simulink model "Voltage_Source_Inverter_fed_Asynchronous_Motor_Drive"  (R2020b)
settings: Solver=VariableStepAuto  StartTime=0.0  StopTime=10  RelTol=1e-3
libraries: powerlib x12, powerlib_meascontrol x1
settings Model: Creator=adima  LastModifiedBy=adima

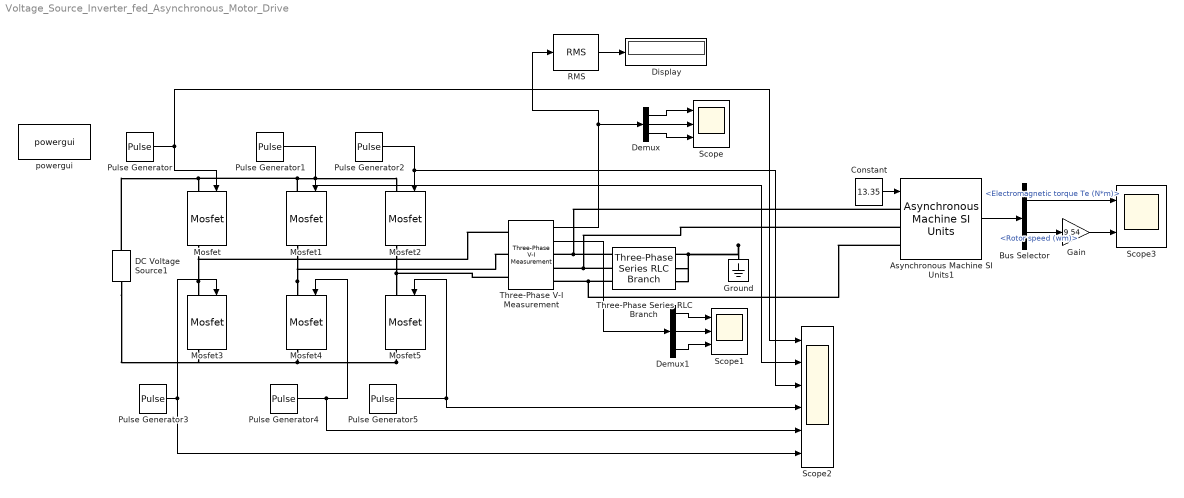
== system Voltage_Source_Inverter_fed_Asynchronous_Motor_Drive ==
  Asynchronous Machine SI Units1 : powerlib/Machines/Asynchronous Machine SI Units  RotorType=Squirrel-cage  PresetModel="15:  5.4 HP (4KW)   400 V  50Hz 1430 RPM"  MechanicalLoad=Torque Tm  ShowDetailedParameters=on  ReferenceFrame=Rotor  Units=SI  MeasurementBus=off  NominalParameters=[4000 400 50]  Stator=[1.405 0.005839]  Rotor=[1.395 0.005839]  Cage1=[0.4155 0.002066]  Cage2=[0.4168 0.0003495]  Lm=0.1722  Mechanical=[0.0131 0.002985 2]  PolePairs=2  InitialConditions=[0 0 0 0 0 0 0 0]  SimulateSaturation=off  Saturation=[14.03593122, 27.81365428, 53.79336849, 72.68890987, 97.98006896, 148.6815601, 215.7428561, 302.9841135, 428.7778367 ; 230, 322, 414, 460, 506, 552, 598, 644, 690]  LoadFlowParameters=1492000  TsPowergui=0  TsBlock=-1  IterativeModel=Trapezoidal non iterative  IterativeDiscreteModel=Trapezoidal non iterative  Pmec=1.492e+006
  Bus Selector : BusSelector  OutputSignals=Mechanical.Electromagnetic torque Te (N*m),Mechanical.Rotor speed (wm)
  Constant : Constant  Value=13.35
  DC Voltage Source1 : powerlib/Electrical Sources/DC Voltage Source  Amplitude=300  Measurements=None
  Demux : Demux  Outputs=3
  Demux1 : Demux  Outputs=3
  Display : Display
  Gain : Gain  Gain=9.54
  Ground : powerlib/Elements/Ground  LConnTagsString=a
  Mosfet{,1..5} (6 alike) : powerlib/Power Electronics/Mosfet  Ron=0.1  Lon=0  Rd=0.01  Vfd=0  IC=0  Rs=1e5  Cs=inf  Measurements=on
  Pulse Generator : DiscretePulseGenerator  PulseType=Time based  Period=1/50  PulseWidth=50
  Pulse Generator1 : DiscretePulseGenerator  PulseType=Time based  Period=1/50  PulseWidth=50  PhaseDelay=120*((20e-3)/360)
  Pulse Generator2 : DiscretePulseGenerator  PulseType=Time based  Period=1/50  PulseWidth=50  PhaseDelay=240*((20e-3)/360)
  Pulse Generator3 : DiscretePulseGenerator  PulseType=Time based  Period=1/50  PulseWidth=50  PhaseDelay=180*((20e-3)/360)
  Pulse Generator4 : DiscretePulseGenerator  PulseType=Time based  Period=1/50  PulseWidth=50  PhaseDelay=300*((20e-3)/360)
  Pulse Generator5 : DiscretePulseGenerator  PulseType=Time based  Period=1/50  PulseWidth=50  PhaseDelay=60*((20e-3)/360)
  RMS : powerlib_meascontrol/Measurements/RMS  TrueRMS=on  Freq=60  RMSInit=120  Ts=0
  Scope : Scope  NumInputPorts=3
  Scope1 : Scope  NumInputPorts=3
  Scope2 : Scope  NumInputPorts=6
  Scope3 : Scope  NumInputPorts=2
  Three-Phase Series RLC Branch : powerlib/Elements/Three-Phase Series RLC Branch  LConnTagsString=A|B|C  RConnTagsString=A|B|C  BranchType=R  Resistance=10  Inductance=1e-3  Capacitance=1e-6  Measurements=None
  Three-Phase V-I Measurement : powerlib/Measurements/Three-Phase V-I Measurement  VoltageMeasurement=phase-to-ground  SetLabelV=off  LabelV=Vabc  Vpu=off  VpuLL=off  CurrentMeasurement=yes  SetLabelI=off  LabelI=Iabc  Ipu=off  Pbase=100e6  Vbase=500e3  OutputType=Complex  PhasorSimulation=off  PSBequivalent=0
  powergui : powerlib/powergui  Priority=1  SimulationMode=Discrete  SampleTime=5e-6  frequency=60  Iterations=50  frequencyindice=0  Pbase=100e6  ErrMax=1e-4  UnitsV=kV  UnitsW=MW  buscounter=0  FunctionMessages=off  echomessages=off  EnableUseOfTLC=off  CurrentSourceSwitches=off  DisableSnubberDevices=off  DisableRonSwitches=off  DisableVfSwitches=off  DisplayEquations=off  AutomaticDiscreteSolvers=off  SolverType=Tustin/Backward Euler (TBE)  Interpol=off  ExternalGateDelay=off  methode=off  Ts=100  x0status=blocks  SPID=on  SwTol=0  HookPort=off  NonlinearTolerance=1e-4  nMaxIteration=100  ContinueOnMaxIteration=off  RestoreLinks=warning  ResistiveCurrentMeasurement=off  Frange=[0:2:500]  Ylog=off  Xlog=on  ShowGrid=off  save=off  variable=ZData  structure=0  ZoomFFT=off  StartTime=0.0  cycles=1  DisplayStyle=1  fundamental=60  FreqAxis=off  MaxFrequency=1000  frequencyindicesteady=1  RmsSteady=1  display=off
  wires:
  Demux1/1 -> Scope1/1
  RMS/1 -> Display/1
  Three-Phase V-I Measurement/2 -> Demux1/1
  Demux/2 -> Scope/2
  Pulse Generator1/1 -> Mosfet1/1, Scope2/2
  Pulse Generator/1 -> Mosfet/1, Scope2/1
  Pulse Generator2/1 -> Scope2/3, Mosfet2/1
  Pulse Generator4/1 -> Scope2/5, Mosfet4/1
  Pulse Generator3/1 -> Scope2/6, Mosfet3/1
  Three-Phase V-I Measurement/1 -> RMS/1, Demux/1
  Pulse Generator5/1 -> Mosfet5/1, Scope2/4
  Demux/1 -> Scope/1
  Demux1/2 -> Scope1/2
  Demux/3 -> Scope/3
  Demux1/3 -> Scope1/3
  Bus Selector/2 -> Gain/1  "<Rotor speed (wm)>"
  Constant/1 -> Asynchronous Machine SI Units1/1
  Asynchronous Machine SI Units1/1 -> Bus Selector/1
  Gain/1 -> Scope3/2
  Bus Selector/1 -> Scope3/1  "<Electromagnetic torque Te (N*m)>"
  connections:
  Ground/LConn1 -- Three-Phase Series RLC Branch/RConn3 -- Three-Phase Series RLC Branch/RConn2 -- Three-Phase Series RLC Branch/RConn1
  Mosfet3/LConn1 -- Mosfet/RConn1 -- Three-Phase V-I Measurement/LConn1
  Mosfet5/RConn1 -- Mosfet4/RConn1 -- DC Voltage Source1/LConn1 -- Mosfet3/RConn1
  Mosfet1/LConn1 -- DC Voltage Source1/RConn1 -- Mosfet/LConn1 -- Mosfet2/LConn1
  Three-Phase V-I Measurement/LConn3 -- Mosfet2/RConn1 -- Mosfet5/LConn1
  Mosfet4/LConn1 -- Mosfet1/RConn1 -- Three-Phase V-I Measurement/LConn2
  Three-Phase Series RLC Branch/LConn1 -- Asynchronous Machine SI Units1/LConn1 -- Three-Phase V-I Measurement/RConn1
  Three-Phase Series RLC Branch/LConn2 -- Asynchronous Machine SI Units1/LConn2 -- Three-Phase V-I Measurement/RConn2
  Three-Phase Series RLC Branch/LConn3 -- Asynchronous Machine SI Units1/LConn3 -- Three-Phase V-I Measurement/RConn3
